simulink model "test_2"  (R2019b)
settings: Solver=VariableStepAuto  StartTime=0.0  StopTime=simTime  RelTol=1e-3
values from neighbouring files (symbols this model uses):
  delta = 1    [tset_1.m]
  den = [1 1]    [tset_1.m]
  num = [1]    [tset_1.m]
settings Model: Creator=朱佳琪  LastModifiedBy=朱佳琪
settings DataIOCC: ReturnWorkspaceOutputs=off

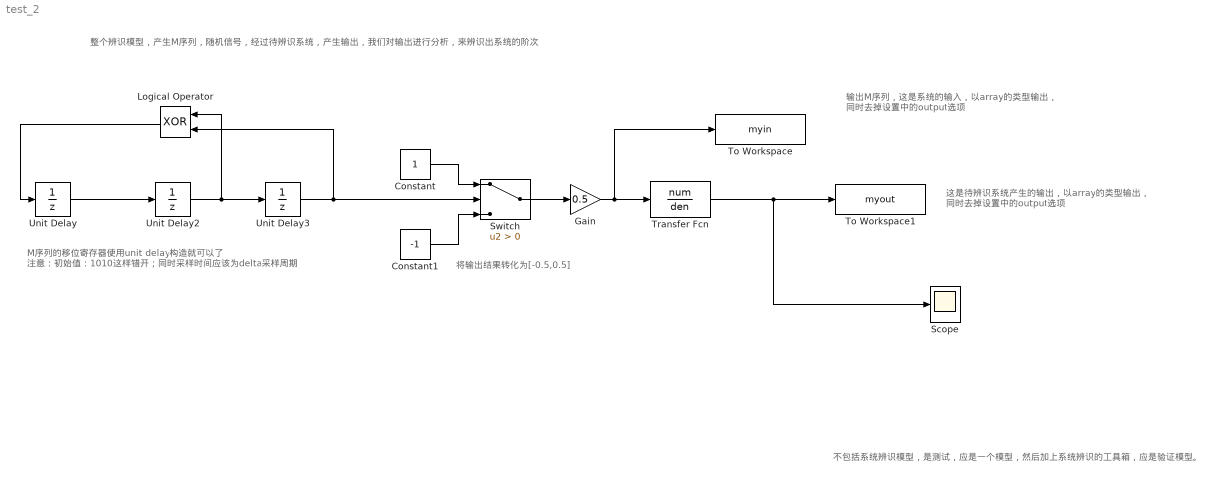
== system test_2 ==
  note: 整个辨识模型，产生M序列，随机信号，经过待辨识系统，产生输出，我们对输出进行分析，来辨识出系统的阶次
  note: 这是待辨识系统产生的输出，以array的类型输出，
      | 同时去掉设置中的output选项
  note: 输出M序列，这是系统的输入，以array的类型输出，
      | 同时去掉设置中的output选项
  note: 将输出结果转化为[-0.5,0.5]
  note: M序列的移位寄存器使用unit delay构造就可以了
      | 注意：初始值：1010这样错开；同时采样时间应该为delta采样周期
  note: 不包括系统辨识模型，是测试，应是一个模型，然后加上系统辨识的工具箱，应是验证模型。
  Constant : Constant
  Constant1 : Constant  Value=-1
  Gain : Gain  Gain=0.5
  Logical Operator : Logic  Operator=XOR  AllPortsSameDT=off  OutDataTypeStr=boolean
  Scope : Scope
  Switch : Switch  Criteria=u2 > Threshold
  To Workspace : ToWorkspace  VariableName=myin  SampleTime=delta
  To Workspace1 : ToWorkspace  VariableName=myout  SampleTime=delta
  Transfer Fcn : TransferFcn  Numerator=num  Denominator=den
  Unit Delay : UnitDelay  SampleTime=delta  HasFrameUpgradeWarning=on
  Unit Delay2 : UnitDelay  InitialCondition=1  SampleTime=delta  HasFrameUpgradeWarning=on
  Unit Delay3 : UnitDelay  SampleTime=delta  HasFrameUpgradeWarning=on
  wires:
  Unit Delay/1 -> Unit Delay2/1
  Unit Delay3/1 -> Switch/2, Logical Operator/2
  Constant/1 -> Switch/1
  Constant1/1 -> Switch/3
  Logical Operator/1 -> Unit Delay/1
  Switch/1 -> Gain/1
  Gain/1 -> Transfer Fcn/1, To Workspace/1
  Transfer Fcn/1 -> Scope/1, To Workspace1/1
  Unit Delay2/1 -> Unit Delay3/1, Logical Operator/1
